simulink library "dynamics"  (R2025b)
settings: Solver=VariableStepAuto  StartTime=0.0  StopTime=10.0  RelTol=1e-3
values from neighbouring files (symbols this model uses):
  I = diag([ ix iy iz ])    [lab_7_task_1.m]    (also in lab_7_task_3.m = diag([ ix iy iz ] * 10^-2))
  w0 = [0.45; 0.52; 0.55;]    [lab_7_task_1.m]    (also in lab_7_task_3.m)
libraries: matrix_library x1
settings Model: Creator=User  LastModifiedBy=nicol

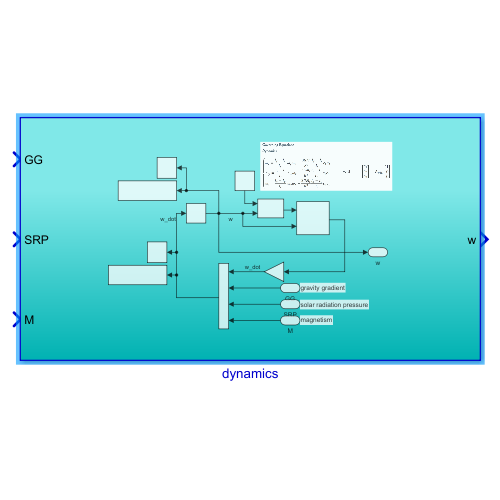
[thumbnail: Simulink's stored preview of the top-level diagram]
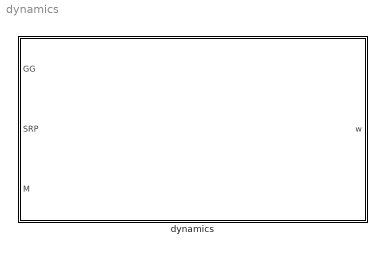
== system dynamics ==
  dynamics : Subsystem

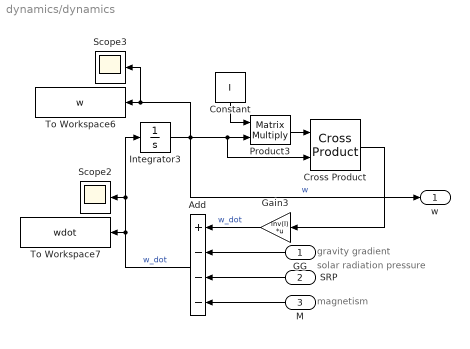
== system dynamics/dynamics ==
  note: magnetism
  note: solar radiation pressure
  note: gravity gradient
  GG : Inport
  SRP : Inport  Port=2
  M : Inport  Port=3
  Add : Sum  Inputs=+---
  Constant : Constant  Value=I
  Cross Product : matrix_library/Cross Product
  Gain3 : Gain  Gain=inv(I)  Multiplication=Matrix(K*u)
  Integrator3 : Integrator  InitialCondition=w0
  Product3 : Product  Multiplication=Matrix(*)
  Scope2 : Scope
      settings: ActiveDisplayYMinimum=-1  ActiveDisplayYMaximum=1  DataLoggingVariableName=ScopeData2
  Scope3 : Scope
      settings: ActiveDisplayYMinimum=-1  ActiveDisplayYMaximum=1  DataLoggingVariableName=ScopeData3
  To Workspace6 : ToWorkspace  VariableName=w  SaveFormat=Timeseries  SampleTime=-1
  To Workspace7 : ToWorkspace  VariableName=wdot  SaveFormat=Timeseries  SampleTime=-1
  w : Outport
  wires:
  Product3/1 -> Cross Product/1
  Add/1 -> Integrator3/1, Scope2/1, To Workspace7/1  "w_dot"
  Cross Product/1 -> Gain3/1
  GG/1 -> Add/2
  Gain3/1 -> Add/1  "w_dot"
  Integrator3/1 -> w/1, Cross Product/2, Product3/2, To Workspace6/1, Scope3/1  "w"
  Constant/1 -> Product3/1
  SRP/1 -> Add/3
  M/1 -> Add/4
